simulink model "BuckConverter"  (R2025b)
settings: Solver=ode23tb  StartTime=0.0  StopTime=120e-3  MaxStep=1e-6  RelTol=1e-5
values from neighbouring files (symbols this model uses):
  d1 = 1.0    (= 1)    [Scenario.m]    (also in Scenario_Perfect.m; optimize_controllers.m)
  d2 = den_3p2z(2) / den_3p2z(1)    [Scenario.m]    (also in Scenario_Perfect.m = -(A_p^2 + 2*A_p) / d_raw1; optimize_controllers.m = d_raw2 / d_raw1)
  d3 = den_3p2z(3) / den_3p2z(1)    [Scenario.m]    (also in Scenario_Perfect.m = (2*A_p + 1) / d_raw1; optimize_controllers.m = d_raw3 / d_raw1)
  K_lqr1 = 0.55    [Scenario.m]    (also in Scenario_Perfect.m = K_lqr_all(1); optimize_controllers.m = K_lqr_all(1))
  K_lqr2 = 1.05    [Scenario.m]    (also in Scenario_Perfect.m = K_lqr_all(2); optimize_controllers.m = K_lqr_all(2))
  K_lqr3 = -8500    [Scenario.m]    (also in Scenario_Perfect.m = K_lqr_all(3); optimize_controllers.m = K_lqr_all(3))
  KI = 500    [Scenario.m]    (also in Scenario_Perfect.m = gbest_pi(2))
  KP = 0.08    [Scenario.m]    (also in Scenario_Perfect.m = gbest_pi(1))
  m1 = m_coeff(1) / e_coeff(1)    [Scenario.m]    (also in Scenario_Perfect.m = m_coeff(1); optimize_controllers.m = m_coeff(1))
  m2 = m_coeff(2) / e_coeff(1)    [Scenario.m]    (also in Scenario_Perfect.m = m_coeff(2); optimize_controllers.m = m_coeff(2))
  m3 = m_coeff(3) / e_coeff(1)    [Scenario.m]    (also in Scenario_Perfect.m = m_coeff(3); optimize_controllers.m = m_coeff(3))
  m4 = m_coeff(4) / e_coeff(1)    [Scenario.m]    (also in Scenario_Perfect.m = m_coeff(4); optimize_controllers.m = m_coeff(4))
  m5 = m_coeff(5) / e_coeff(1)    [Scenario.m]    (also in Scenario_Perfect.m = m_coeff(5); optimize_controllers.m = m_coeff(5))
  n1 = num_3p2z(1) / den_3p2z(1)    [Scenario.m]    (also in Scenario_Perfect.m = (K_c * T_s * A_z^2) / d_raw1; optimize_controllers.m = n_raw1 / d_raw1)
  n2 = num_3p2z(2) / den_3p2z(1)    [Scenario.m]    (also in Scenario_Perfect.m = (-2 * K_c * T_s * A_z) / d_raw1; optimize_controllers.m = n_raw2 / d_raw1)
  n3 = num_3p2z(3) / den_3p2z(1)    [Scenario.m]    (also in Scenario_Perfect.m = (K_c * T_s) / d_raw1; optimize_controllers.m = n_raw3 / d_raw1)
  Ts = T_s    (= 1e-05)    [Scenario.m]    (also in Scenario_Perfect.m; Scenario_Perfect_Final.m)
undefined symbols (not defined in the file or in its folder): DiscIntNeverNeededParam, dspblkCoreblockFVToolHelper, gcbh
libraries: nesl_utility x32, fl_lib x24, ee_lib x12, eePwmGenerator x4, slpidlib x1, mpclib x1
settings Model: Creator=vivid  LastModifiedBy=vivid

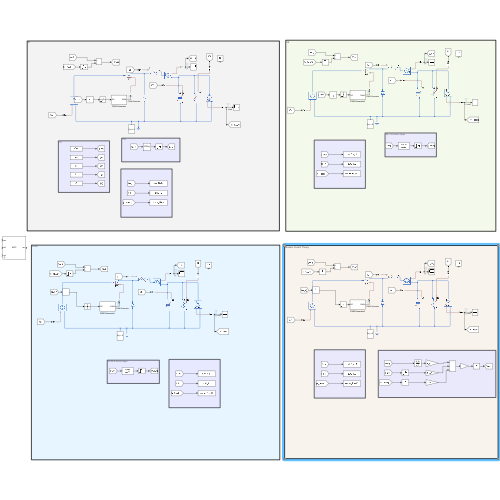
[thumbnail: Simulink's stored preview of the top-level diagram]
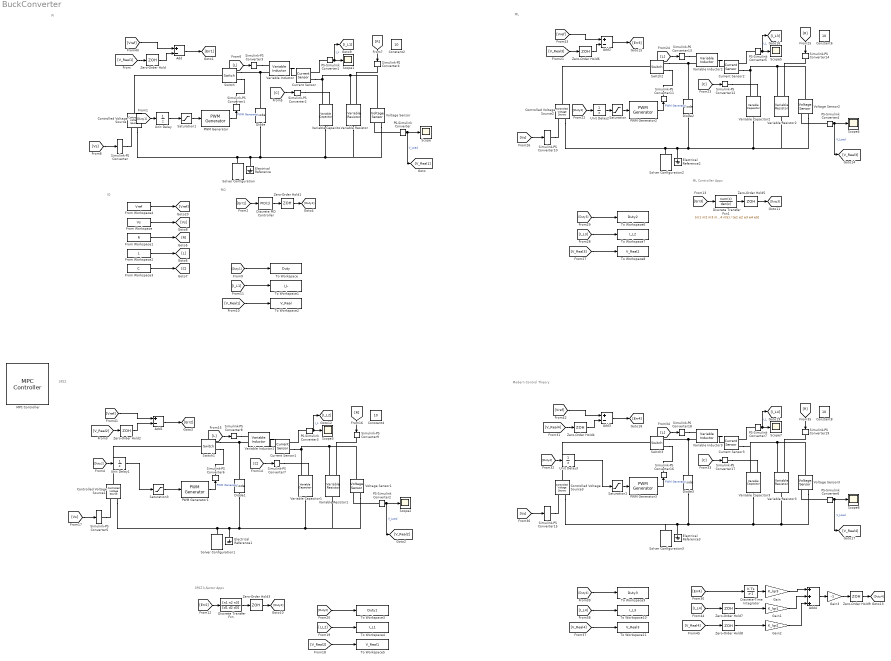
== system BuckConverter ==
  note: Modern Control Theory
  note: ML
  note: 3P2Z
  note: PI
  note: IO
  note: PID
  note: ML Controller Appx
  note: 3P2Z k-factor Appx
  Add{,1..3} (4 alike) : Sum  Inputs=+-
  Add4 : Sum  Inputs=+++
  Constant{2,4,6,8} (4 alike) : Constant  Value=10
  Controlled Voltage Source{,1..3} (4 alike) : fl_lib/Electrical/Electrical Sources/Controlled Voltage Source
  Current Sensor{,1..3} (4 alike) : fl_lib/Electrical/Electrical Sensors/Current Sensor
  Diode{,1..3} (4 alike) : ee_lib/Semiconductors & Converters/Diode  ModelType=ee.enum.diode.modelType.pwl  TableType=ee.enum.diode.tableType.IfMat  IfMat=[.07, .12, .19, 1.75, 4.24, 7.32, 11.2; .16, .3, .72, 2.14, 5.02, 8.35, 13.12] A  VfMat=[.9, 1.15, 1.25, 1.5, 1.75, 2.17, 2.6, 2.85; .58, .68, .75, 1.1, 1.38, 1.77, 2.27, 2.7] V  TjVec=[25, 125] degC  VfVec=[.5, .7, .9, 1.3, 1.7, 2.1, 2.5] V  IfVec=[.1, .2, .5, 1, 2, 4, 7, 10] A  IrMat=[1e-06, 2e-06, 5e-06, 1e-05, 2.5e-05, 5e-05, .0001; 2e-06, 5e-06, 1e-05, 4e-05, 8e-05, .0002, .0005] A  VrMat=[10, 100, 200, 250, 300, 325, 350; 10, 70, 160, 220, 270, 300, 320] V  VrVec=[10, 20, 40, 50, 70, 80, 100] V  IrVec=[1e-06, 2e-06, 5e-06, 1e-05, 2e-05, 5e-05, .0001] A  Vf=0.6 V  Ron=0.3 Ohm  Goff=1e-8 S  prmExp=ee.enum.diode.expParam.useTwo  I12=[.0137, .545] A  V12=[.6, .7] V  RS=0 Ohm  Tmeas=298.15 K  IS=1e-12 A  ec=1  I1=0.0137 A  V1=0.6 V  N_series=1  N_parallel=1  ZenerEnable=false  Rz=0.3 Ohm  BV=inf V  C_param=ee.enum.diode.capParam.fixed  CJ=0 pF  CJ0=5 pF  Vvec=[.1, 10, 100] V  Cvec=[3.5, 1, .4] pF  VJ=1 V  Mgrad=0.5  FC=0.5  Q_param=ee.enum.diode.recoveryParam.off  iRM=-7.15 A  iF=4 A  didt=-750 A/us  trr_factor=3  trr=115 ns  Qrr=150 nA*s  Vr=-600 V  Ls=150 nH  Erec=0.03 J  TT=50 ns  tau=100 ns  T_param=ee.enum.diode.temperatureParam.off  Tdevice=298.15 K  I1_T2=0.245 A  V1_T2=0.5 V  IS_T2=1.25e-7 A  Tmeas2=125 degC  XTI_param=ee.enum.diode.xtiParam.pn  XTI=3  EG_param=ee.enum.diode.egapParam.material_si  EG=1.11 eV  dBVdT=0 V/K  enable_fault_input=simscape.enum.onoff.off  i_specify=off  i_priority=None  i=0 A  i_nominal_specify=off  i_nominal_value=1  i_nominal_unit=A  v_specify=off  v_priority=None  v=0 V  v_nominal_specify=off  v_nominal_value=1  v_nominal_unit=V  v_capacitor_specify=off  v_capacitor_priority=None  v_capacitor=0 V  v_capacitor_nominal_specify=off  v_capacitor_nominal_value=1  v_capacitor_nominal_unit=V  Qj_specify=off  Qj_priority=High  Qj=0 C  Qj_nominal_specify=off  Qj_nominal_value=1  Qj_nominal_unit=C  i_diode_specify=off  i_diode_priority=None  i_diode=0 A  i_diode_nominal_specify=off  i_diode_nominal_value=1  i_diode_nominal_unit=A  v_diode_specify=off  v_diode_priority=None  v_diode=0 V  v_diode_nominal_specify=off  v_diode_nominal_value=1  v_diode_nominal_unit=V  i_capacitor_specify=off  i_capacitor_priority=None  i_capacitor=0 A  i_capacitor_nominal_specify=off  i_capacitor_nominal_value=1  i_capacitor_nominal_unit=A  power_dissipated_specify=off  power_dissipated_priority=None  power_dissipated=0 W  power_dissipated_nominal_specify=off  power_dissipated_nominal_value=1  power_dissipated_nominal_unit=W  fidelity_level=ee.enum.diode.fidelity.includeChargeDyn  rec_loss_model=ee.enum.diode.reverseRecoveryModel.fixed  ErecVal=0 J  scaleWithIandV=true  ErecMat=zeros(2, 3) J  TjrecVec=[298.15, 398.15] K  IfrecVec=[.1, 1, 10] A  IrecVal=10 A  VrecVal=10 V  tFilter=1 / 1000 / 100 s  thermal_network_parameterization=ee.enum.thermalNetworkTopology.junctionCase  Rth=[0, 10] K/W  Rth_Cauer=[1, 3, 10] K/W  Rth_Foster=[.08, .14, .22, .16] K/W  thermal_mass_parameterization=ee.enum.thermalNetwork.timeconstant  thermal_mass=[0, 1] J/K  thermal_mass_Cauer=[.1, .3, 1] J/K  thermal_mass_Foster=[.001, .005, .05, .5] J/K  thermal_time_constant=[0, 10] s  thermal_time_constant_Cauer=[1, 3, 10] s  thermal_time_constant_Foster=[7e-05, .0007, .01, .08] s  thermal_mass_initial_temperatures=[25, 25] degC  thermal_mass_initial_temperatures_Cauer=[25, 25, 25] degC  junction_thermal_mass=0.01 J/K  Tvec_initial_Foster=[25, 25, 25, 25] degC  no_thermal_network=0  junction_temperature_specify=off  junction_temperature_priority=None  junction_temperature=25 degC  junction_temperature_nominal_specify=off  junction_temperature_nominal_value=1  junction_temperature_nominal_unit=degC
  Discrete Transfer Fcn : DiscreteTransferFcn  LoadFcn=dspblkCoreblockFVToolHelper(gcbh,'load');  Numerator=[n1 n2 n3]  Denominator=[d1 d2 d3]
      settings: CopyFcn=dspblkCoreblockFVToolHelper(gcbh,'copy');  DeleteFcn=dspblkCoreblockFVToolHelper(gcbh,'close');  ModelCloseFcn=dspblkCoreblockFVToolHelper(gcbh,'close');  PreSaveFcn=dspblkCoreblockFVToolHelper(gcbh,'presave');  PostSaveFcn=dspblkCoreblockFVToolHelper(gcbh,'postsave');  CloseFcn=dspblkCoreblockFVToolHelper(gcbh,'close');
  Discrete Transfer Fcn1 : DiscreteTransferFcn  LoadFcn=dspblkCoreblockFVToolHelper(gcbh,'load');  Numerator=[m1 m2 m3 m4 m5]  Denominator=[e1 e2 e3 e4 e5]
      settings: CopyFcn=dspblkCoreblockFVToolHelper(gcbh,'copy');  DeleteFcn=dspblkCoreblockFVToolHelper(gcbh,'close');  ModelCloseFcn=dspblkCoreblockFVToolHelper(gcbh,'close');  PreSaveFcn=dspblkCoreblockFVToolHelper(gcbh,'presave');  PostSaveFcn=dspblkCoreblockFVToolHelper(gcbh,'postsave');  CloseFcn=dspblkCoreblockFVToolHelper(gcbh,'close');
  Discrete PID Controller : slpidlib/PID Controller  Controller=PID  Form=Parallel  TimeDomain=Discrete-time  UseExternalTs=off  SampleTime=Ts  IntegratorMethod=Forward Euler  FilterMethod=Forward Euler  ControllerParametersSource=internal  P=KP  I=KI  UseKiTs=off  D=0  UseExternalDerivativeSource=off  N=100  UseFilter=on  TunerSelectOption=Transfer Function Based (PID Tuner App)  InitialConditionSource=internal  InitialConditionForIntegrator=0  InitialConditionForFilter=0  DifferentiatorICPrevScaledInput=0  ExternalReset=none  TrackingMode=off  Kt=1  LimitOutput=off  SatLimitsSource=internal  UpperSaturationLimit=inf  LowerSaturationLimit=-inf  LinearizeAsGain=off  AntiWindupMode=none  Kb=1  LimitIntegrator=off  UpperIntegratorSaturationLimit=inf  LowerIntegratorSaturationLimit=-inf  POutMin=[]  POutMax=[]  IOutMin=[]  IOutMax=[]  DOutMin=[]  DOutMax=[]  NOutMin=[]  NOutMax=[]  SumOutMin=[]  SumOutMax=[]  SaturationOutMin=[]  SaturationOutMax=[]  PParamMin=[]  PParamMax=[]  IParamMin=[]  IParamMax=[]  DParamMin=[]  DParamMax=[]  NParamMin=[]  NParamMax=[]  KbParamMin=[]  KbParamMax=[]  KtParamMin=[]  KtParamMax=[]  KbOutMin=[]  KbOutMax=[]  KtOutMin=[]  KtOutMax=[]  IntegratorOutMin=[]  IntegratorOutMax=[]  FilterOutMin=[]  FilterOutMax=[]  SumI1OutMin=[]  SumI1OutMax=[]  SumI2OutMin=[]  SumI2OutMax=[]  SumI3OutMin=[]  SumI3OutMax=[]  SumI4OutMin=[]  SumI4OutMax=[]  SumDOutMin=[]  SumDOutMax=[]  DifferentiatorOutMin=[]  DifferentiatorOutMax=[]  FilterDiffOutCoefMin=[]  FilterDiffOutCoefMax=[]  ReciprocalOutMin=[]  ReciprocalOutMax=[]  SumDenOutMin=[]  SumDenOutMax=[]  SumNumOutMin=[]  SumNumOutMax=[]  DivideOutMin=[]  DivideOutMax=[]  UdiffTsProdOutMin=[]  UdiffTsProdOutMax=[]  NTsProdOutMin=[]  NTsProdOutMax=[]  UintegralTsProdOutMin=[]  UintegralTsProdOutMax=[]  UngainTsProdOutMin=[]  UngainTsProdOutMax=[]  ClampingZeroOutDataTypeStr=Inherit: Inherit via back propagation  ClampingZeroOutMin=[]  ClampingZeroOutMax=[]  FilterDenConstantOutDataTypeStr=Inherit: Inherit via back propagation  FilterDenConstantOutMin=[]  FilterDenConstantOutMax=[]  PCopyOutDataTypeStr=Inherit: Inherit via back propagation  PCopyOutMin=[]  PCopyOutMax=[]  NCopyOutDataTypeStr=Inherit: Inherit via back propagation  NCopyOutMin=[]  NCopyOutMax=[]  IntegratorContinuousStateAttributes=''  IntegratorStateMustResolveToSignalObject=off  IntegratorRTWStateStorageClass=Auto  FilterContinuousStateAttributes=''  FilterStateMustResolveToSignalObject=off  FilterRTWStateStorageClass=Auto  ParallelPVariant=InternalParameters  IdealPVariant=Disabled  IVariant=InternalParameters  DVariant=InternalParameters  IntegratorVariant=Discrete  SatVariant=Disabled  AWVariant=Passthrough  PCopyVariant=Disabled  TRVariant=Disabled  FdbkBlocksVariant=Forward  IdealPFdbkVariant=Disabled  SatFdbkVariant=Disabled  DerivativeFilterVariant=ForwardEulerFilter  NVariant=InternalParameters  NCopyVariant=Disabled  FilterICVariant=InternalICsFilter  IntegratorICVariant=InternalICs  ExternalResetVariant=Disabled  TRSumVariant=Passthrough  SumFdbkVariant=Disabled  SumVariant=Sum_PID  TsampFilterVariant=InternalTs  TsampNgainVariant=Passthrough  TsampIntegralVariant=Disabled_SignalSpec  ExternalSaturationOutDataTypeStr=Inherit: Same as second input  DerivativeSourceVariant=ErrorSignal  PreIntVariant=InternalPreInt
      settings: LibrarySourceBlock=simulink/Discrete/Discrete PID Controller
  Discrete-Time Integrator : DiscreteIntegrator  SampleTime=Ts  ICPrevOutput=DiscIntNeverNeededParam  ICPrevScaledInput=DiscIntNeverNeededParam
  Electrical Reference{,1..3} (4 alike) : fl_lib/Electrical/Electrical Elements/Electrical Reference
  From Workspace : FromWorkspace  VariableName=Vs
  From Workspace1 : FromWorkspace  VariableName=R
  From Workspace2 : FromWorkspace  VariableName=L
  From Workspace3 : FromWorkspace  VariableName=C
  From Workspace4 : FromWorkspace  VariableName=Vref
  Gain : Gain  Gain=K_lqr3
  Gain1 : Gain  Gain=K_lqr1
  Gain2 : Gain  Gain=K_lqr2
  Gain3 : Gain  Gain=-1
  MPC Controller : mpclib/MPC Controller  SCDEnableBlockLinearizationSpecification=on  is_multiple=0  enable_value=0  return_u0=off  updateMPCinCallerWorkspace=on  md_inport=on  mv_inport=off  uref_inport=off  return_cost=off  return_mvseq=off  return_qpstatus=off  return_xseq=off  return_state=off  return_ovseq=off  state_inport=off  umin_inport=off  umax_inport=off  ymin_inport=off  ymax_inport=off  cc_inport=off  ywt_inport=off  uwt_inport=off  duwt_inport=off  rhoeps_inport=off  pm_inport=off  MaximumP=10  HorizonChoice=FixedHorizon  n_ts=1  n_p=10  n_mv=1  n_md=1  n_ud=0  n_mo=1  n_uo=0  BlockDataType=double  SampleTimeInherited=off  switch_inport=off
  PS-Simulink Converter{,1..7} (8 alike) : nesl_utility/PS-Simulink Converter  PhysicalDomain=network_engine_domain  SubClassName=ps_output  LeftPortType=input  RightPortType=output  PseudoPeriodic=off  Frequencies=[]  VectorFormat=inherit  Unit=inherit  AffineConversion=off
  PWM Generator{,1..3} (4 alike) : eePwmGenerator/PWM Generator  CarrCount=Up  Tper=Ts  Tdelay=0  Ts=1e-7
  Saturation{,1..3} (4 alike) : Saturate  UpperLimit=0.95  LowerLimit=0.01
  Scope{,1..7} (8 alike) : Scope
      Scope2 settings: DataLoggingVariableName=ScopeData2
      Scope3 settings: DataLoggingVariableName=ScopeData3
      Scope4 settings: DataLoggingVariableName=ScopeData4
      Scope5 settings: DataLoggingVariableName=ScopeData5
      Scope6 settings: DataLoggingVariableName=ScopeData6
      Scope7 settings: DataLoggingVariableName=ScopeData7
  Simulink-PS Converter{,4..5,9..10,14..15,19} (8 alike) : nesl_utility/Simulink-PS Converter  PhysicalDomain=network_engine_domain  SubClassName=ps_input  LeftPortType=input  RightPortType=output  PseudoPeriodic=off  Frequencies=[]  NoiseDistribution=none  NoiseParameters=[]  Unit=1  AffineConversion=off  FilteringAndDerivatives=filter  SimscapeFilterOrder=1  InputFilterTimeConstant=0.001  UdotUserProvided=0
  Simulink-PS Converter{1..3,6..8,11..13,16..18} (12 alike) : nesl_utility/Simulink-PS Converter  PhysicalDomain=network_engine_domain  SubClassName=ps_input  LeftPortType=input  RightPortType=output  PseudoPeriodic=off  Frequencies=[]  NoiseDistribution=none  NoiseParameters=[]  Unit=1  AffineConversion=off  FilteringAndDerivatives=provide  SimscapeFilterOrder=1  InputFilterTimeConstant=0.001  UdotUserProvided=0
  Solver Configuration{,1..3} (4 alike) : nesl_utility/Solver Configuration  PhysicalDomain=network_engine_domain  SubClassName=solver  LeftPortType=input  RightPortType=generic  Tones=[]  Harmonics=[]  SimulateNoise=off  Profile=off  UseLocalSampling=off  EnableSwitchedLinearOptims=on  FrequencyDomain=off  UseCCode=off  RelTol=0.001  AbsTol=0.001  MinStep=1e-09  ToWorkspace=off  RevertToSquareIcSolve=off  NumHomotopyIterations=100  PhasorMode=off  PhasorModeNumHarmonics=1  ConsistencySolver=NEWTON_XTOL_AFTER_FTOL  IndexReductionMethod=DerivativeReplacement  DoDC=off  ResidualTolerance=1e-09  ConsistencyTolSource=GLOBAL  ConsistencyAbsTol=0.001  ConsistencyRelTol=0.001  ConsistencyTolFactor=0.001  UseLocalSolver=off  LocalSolverChoice=NE_BACKWARD_EULER_ADVANCER  ResolveIndetEquations=on  FunctionEvalNumThread=1  LocalSolverSampleTime=0.001  DoFixedCost=off  MaxNonlinIter=3  MaxModeIter=2  ComputeImpulses=off  ImpulseIterations=2  LinearAlgebra=auto  LinearAlgebraNumThread=0  EquationFormulation=NE_TIME_EF  DelaysMemoryBudget=1024  AutomaticFiltering=on  FilteringTimeConstant=0.001  PartitionStorageMethod=AS_NEEDED  PartitionMemoryBudget=1024  PartitionMethod=ROBUST  MultibodyUseLocalSolver=off  MultibodyLocalSolverChoice=ODE1  MultibodyLocalSolverSampleTime=0.001
  Switch{,1..3} (4 alike) : fl_lib/Electrical/Electrical Elements/Switch  R_closed=0.01 Ohm  G_open=1e-8 1/Ohm  Threshold=0.5  i_specify=off  i_priority=None  i=0 A  i_nominal_specify=off  i_nominal_value=1  i_nominal_unit=A  v_specify=off  v_priority=None  v=0 V  v_nominal_specify=off  v_nominal_value=1  v_nominal_unit=V
  To Workspace : ToWorkspace  VariableName=Duty  SaveFormat=Timeseries  SampleTime=-1
  To Workspace1 : ToWorkspace  VariableName=I_L  SaveFormat=Timeseries  SampleTime=-1
  To Workspace10 : ToWorkspace  VariableName=I_L3  SaveFormat=Timeseries  SampleTime=-1
  To Workspace11 : ToWorkspace  VariableName=V_Real3  SaveFormat=Timeseries  SampleTime=-1
  To Workspace2 : ToWorkspace  VariableName=V_Real  SaveFormat=Timeseries  SampleTime=-1
  To Workspace3 : ToWorkspace  VariableName=Duty1  SaveFormat=Timeseries  SampleTime=-1
  To Workspace4 : ToWorkspace  VariableName=I_L1  SaveFormat=Timeseries  SampleTime=-1
  To Workspace5 : ToWorkspace  VariableName=V_Real1  SaveFormat=Timeseries  SampleTime=-1
  To Workspace6 : ToWorkspace  VariableName=Duty2  SaveFormat=Timeseries  SampleTime=-1
  To Workspace7 : ToWorkspace  VariableName=I_L2  SaveFormat=Timeseries  SampleTime=-1
  To Workspace8 : ToWorkspace  VariableName=V_Real2  SaveFormat=Timeseries  SampleTime=-1
  To Workspace9 : ToWorkspace  VariableName=Duty3  SaveFormat=Timeseries  SampleTime=-1
  Unit Delay{,1..3} (4 alike) : UnitDelay  SampleTime=-1  HasFrameUpgradeWarning=on
  Variable Capacitor{,1..3} (4 alike) : ee_lib/Passive/Variable Capacitor  prm=2  Cmin=1e-9 F  r=0.05 Ohm  v0=0 V  q0=0 C
      settings: InternalSimscapePortConfiguration="{\"Bottom\":[],\"Left\":[{\"id\":\"C\",\"label\":\"C\",\"type\":\"input\"},{\"id\":\"p\",\"label\":\"+\",\"type\":\"foundation.electrical.electrical\"}],\"Right\":[{\"id\":\"n\",\"label\":\"-\",\"type\":\"foundation.electrical.electrical\"}],\"Top\":[]}"
  Variable Inductor{,1..3} (4 alike) : ee_lib/Passive/Variable Inductor  prm=2  Lmin=1e-6 H  g=1e-3 1/Ohm  i0=0 A  phi0=0 Wb
      settings: InternalSimscapePortConfiguration="{\"Bottom\":[],\"Left\":[{\"id\":\"L\",\"label\":\"L\",\"type\":\"input\"},{\"id\":\"p\",\"label\":\"+\",\"type\":\"foundation.electrical.electrical\"}],\"Right\":[{\"id\":\"n\",\"label\":\"-\",\"type\":\"foundation.electrical.electrical\"}],\"Top\":[]}"
  Variable Resistor{,1..3} (4 alike) : fl_lib/Electrical/Electrical Elements/Variable Resistor  Rmin=0 Ohm  thermalEnable=false  thermal_mass=1 J/K  i_specify=off  i_priority=None  i=0 A  i_nominal_specify=off  i_nominal_value=1  i_nominal_unit=A  v_specify=off  v_priority=None  v=0 V  v_nominal_specify=off  v_nominal_value=1  v_nominal_unit=V  T_specify=off  T_priority=None  T=300 K  T_nominal_specify=off  T_nominal_value=1  T_nominal_unit=K
  Voltage Sensor{,1..3} (4 alike) : fl_lib/Electrical/Electrical Sensors/Voltage Sensor
  Zero-Order Hold{,1..9} (10 alike) : ZeroOrderHold  SampleTime=Ts
  wires:
  PS-Simulink Converter/1 -> [V_Real1], Scope/1  "V_Load"
  PS-Simulink Converter1/1 -> [I_L1], Scope1/1  "I_L"
  [Duty1] -> Unit Delay/1
  PWM Generator/1 -> Simulink-PS Converter1/1  "PWM Generator"
  [Vref] -> Add/1
  [V_Real1] -> Zero-Order Hold/1
  Add/1 -> [Err1]
  [Vs] -> Simulink-PS Converter/1
  [Err1] -> Discrete PID Controller/1
  Discrete PID Controller/1 -> Zero-Order Hold1/1
  [C] -> Simulink-PS Converter2/1
  [L] -> Simulink-PS Converter3/1
  [R] -> Simulink-PS Converter4/1
  From Workspace3/1 -> [C]
  From Workspace2/1 -> [L]
  From Workspace1/1 -> [R]
  From Workspace/1 -> [Vs]
  [Duty1] -> To Workspace/1
  [I_L1] -> To Workspace1/1
  [V_Real1] -> To Workspace2/1
  [Err3] -> Discrete Transfer Fcn1/1
  Discrete Transfer Fcn1/1 -> Zero-Order Hold5/1
  Discrete Transfer Fcn/1 -> Zero-Order Hold3/1
  [Err2] -> Discrete Transfer Fcn/1
  Unit Delay/1 -> Saturation1/1
  Unit Delay1/1 -> Saturation3/1
  [R] -> Simulink-PS Converter9/1
  [L] -> Simulink-PS Converter8/1
  [C] -> Simulink-PS Converter7/1
  [Vs] -> Simulink-PS Converter5/1
  Add1/1 -> [Err2]
  [V_Real2] -> Zero-Order Hold2/1
  [Vref] -> Add1/1
  PWM Generator1/1 -> Simulink-PS Converter6/1  "PWM Generator"
  [Duty2] -> Unit Delay1/1
  PS-Simulink Converter3/1 -> Scope3/1, [I_L2]  "I_L"
  PS-Simulink Converter2/1 -> Scope2/1, [V_Real2]  "V_Load"
  [V_Real2] -> To Workspace5/1
  [I_L2] -> To Workspace4/1
  [Duty2] -> To Workspace3/1
  Unit Delay2/1 -> Saturation/1
  [R] -> Simulink-PS Converter14/1
  [L] -> Simulink-PS Converter13/1
  [C] -> Simulink-PS Converter12/1
  [Vs] -> Simulink-PS Converter10/1
  Add2/1 -> [Err3]
  [V_Real3] -> Zero-Order Hold6/1
  [Vref] -> Add2/1
  PWM Generator2/1 -> Simulink-PS Converter11/1  "PWM Generator"
  [Duty3] -> Unit Delay2/1
  PS-Simulink Converter5/1 -> Scope5/1, [I_L3]  "I_L"
  PS-Simulink Converter4/1 -> Scope4/1, [V_Real3]  "V_Load"
  [V_Real3] -> To Workspace8/1
  [I_L3] -> To Workspace7/1
  [Duty3] -> To Workspace6/1
  [Duty4] -> To Workspace9/1
  [I_L4] -> To Workspace10/1
  [V_Real4] -> To Workspace11/1
  PS-Simulink Converter6/1 -> [V_Real4], Scope6/1  "V_Load"
  PS-Simulink Converter7/1 -> [I_L4], Scope7/1  "I_L"
  [Duty4] -> Unit Delay3/1
  PWM Generator3/1 -> Simulink-PS Converter16/1  "PWM Generator"
  [Vref] -> Add3/1
  [V_Real4] -> Zero-Order Hold4/1
  Add3/1 -> [Err4]
  [Vs] -> Simulink-PS Converter15/1
  [C] -> Simulink-PS Converter17/1
  [L] -> Simulink-PS Converter18/1
  [R] -> Simulink-PS Converter19/1
  Unit Delay3/1 -> Saturation2/1
  Add4/1 -> Gain3/1
  [Err4] -> Discrete-Time Integrator/1
  From Workspace4/1 -> [Vref]
  Discrete-Time Integrator/1 -> Gain/1
  [I_L4] -> Zero-Order Hold7/1
  [V_Real4] -> Zero-Order Hold8/1
  Gain/1 -> Add4/1
  Gain1/1 -> Add4/2
  Gain2/1 -> Add4/3
  Gain3/1 -> Zero-Order Hold9/1
  Zero-Order Hold/1 -> Add/2
  Zero-Order Hold1/1 -> [Duty1]
  Zero-Order Hold2/1 -> Add1/2
  Zero-Order Hold3/1 -> [Duty2]
  Zero-Order Hold4/1 -> Add3/2
  Zero-Order Hold6/1 -> Add2/2
  Zero-Order Hold5/1 -> [Duty3]
  Zero-Order Hold7/1 -> Gain1/1
  Zero-Order Hold8/1 -> Gain2/1
  Zero-Order Hold9/1 -> [Duty4]
  Saturation/1 -> PWM Generator2/1
  Saturation1/1 -> PWM Generator/1
  Saturation3/1 -> PWM Generator1/1
  Saturation2/1 -> PWM Generator3/1
  connections:
  Simulink-PS Converter/RConn1 -- Controlled Voltage Source/RConn1
  Controlled Voltage Source/RConn2 -- Solver Configuration/RConn1 -- Electrical Reference/LConn1 -- Variable Capacitor/RConn1 -- Voltage Sensor/RConn2 -- Variable Resistor/RConn1 -- Diode/LConn1
  Switch/LConn1 -- Controlled Voltage Source/LConn1
  Diode/RConn1 -- Switch/RConn2 -- Variable Inductor/LConn2
  Current Sensor/RConn2 -- Variable Capacitor/LConn2 -- Voltage Sensor/LConn1 -- Variable Resistor/LConn2
  Switch/RConn1 -- Simulink-PS Converter1/RConn1
  PS-Simulink Converter/LConn1 -- Voltage Sensor/RConn1
  Variable Inductor/RConn1 -- Current Sensor/LConn1
  PS-Simulink Converter1/LConn1 -- Current Sensor/RConn1
  Simulink-PS Converter4/RConn1 -- Variable Resistor/LConn1
  Simulink-PS Converter3/RConn1 -- Variable Inductor/LConn1
  Simulink-PS Converter2/RConn1 -- Variable Capacitor/LConn1
  Controlled Voltage Source1/RConn2 -- Diode1/LConn1 -- Variable Resistor1/RConn1 -- Voltage Sensor1/RConn2 -- Variable Capacitor1/RConn1 -- Electrical Reference1/LConn1 -- Solver Configuration1/RConn1
  Diode1/RConn1 -- Variable Inductor1/LConn2 -- Switch1/RConn2
  Current Sensor1/RConn2 -- Variable Resistor1/LConn2 -- Voltage Sensor1/LConn1 -- Variable Capacitor1/LConn2
  Simulink-PS Converter7/RConn1 -- Variable Capacitor1/LConn1
  Simulink-PS Converter8/RConn1 -- Variable Inductor1/LConn1
  Simulink-PS Converter9/RConn1 -- Variable Resistor1/LConn1
  PS-Simulink Converter3/LConn1 -- Current Sensor1/RConn1
  PS-Simulink Converter2/LConn1 -- Voltage Sensor1/RConn1
  Switch1/LConn1 -- Controlled Voltage Source1/LConn1
  Switch1/RConn1 -- Simulink-PS Converter6/RConn1
  Simulink-PS Converter5/RConn1 -- Controlled Voltage Source1/RConn1
  Variable Inductor1/RConn1 -- Current Sensor1/LConn1
  Controlled Voltage Source2/RConn2 -- Diode2/LConn1 -- Variable Resistor2/RConn1 -- Voltage Sensor2/RConn2 -- Variable Capacitor2/RConn1 -- Electrical Reference2/LConn1 -- Solver Configuration2/RConn1
  Diode2/RConn1 -- Variable Inductor2/LConn2 -- Switch2/RConn2
  Current Sensor2/RConn2 -- Variable Resistor2/LConn2 -- Voltage Sensor2/LConn1 -- Variable Capacitor2/LConn2
  Simulink-PS Converter12/RConn1 -- Variable Capacitor2/LConn1
  Simulink-PS Converter13/RConn1 -- Variable Inductor2/LConn1
  Simulink-PS Converter14/RConn1 -- Variable Resistor2/LConn1
  PS-Simulink Converter5/LConn1 -- Current Sensor2/RConn1
  PS-Simulink Converter4/LConn1 -- Voltage Sensor2/RConn1
  Switch2/LConn1 -- Controlled Voltage Source2/LConn1
  Switch2/RConn1 -- Simulink-PS Converter11/RConn1
  Simulink-PS Converter10/RConn1 -- Controlled Voltage Source2/RConn1
  Variable Inductor2/RConn1 -- Current Sensor2/LConn1
  Variable Resistor3/RConn1 -- Controlled Voltage Source3/RConn2 -- Solver Configuration3/RConn1 -- Electrical Reference3/LConn1 -- Diode3/LConn1 -- Variable Capacitor3/RConn1 -- Voltage Sensor3/RConn2
  Variable Inductor3/LConn2 -- Diode3/RConn1 -- Switch3/RConn2
  Variable Resistor3/LConn2 -- Current Sensor3/RConn2 -- Variable Capacitor3/LConn2 -- Voltage Sensor3/LConn1
  Variable Inductor3/RConn1 -- Current Sensor3/LConn1
  Simulink-PS Converter15/RConn1 -- Controlled Voltage Source3/RConn1
  Switch3/RConn1 -- Simulink-PS Converter16/RConn1
  Switch3/LConn1 -- Controlled Voltage Source3/LConn1
  Simulink-PS Converter19/RConn1 -- Variable Resistor3/LConn1
  Simulink-PS Converter17/RConn1 -- Variable Capacitor3/LConn1
  PS-Simulink Converter6/LConn1 -- Voltage Sensor3/RConn1
  Simulink-PS Converter18/RConn1 -- Variable Inductor3/LConn1
  PS-Simulink Converter7/LConn1 -- Current Sensor3/RConn1
